simulink subsystem "BallAndPlate_transfer_function_model"  (R2024b)
settings: Solver=VariableStepAuto  StartTime=0.0  StopTime=10.0  RelTol=1e-3
libraries: cstblocks x2
settings Model: Creator=tshintai  LastModifiedBy=tshintai
settings OptimizationCC: ReuseModelBlockBuffer=off
settings DebuggingCC: UnconnectedInputMsg=warning  UnconnectedOutputMsg=warning  UnconnectedLineMsg=warning
settings ModelReferenceCC: EnableRefExpFcnMdlSchedulingChecks=on
settings RTWCC: GPUComputeCapability=3.5  DLArmComputeVersion=19.05

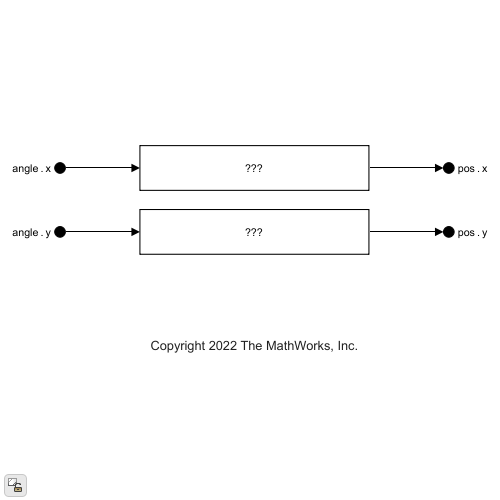
[thumbnail: Simulink's stored preview of the top-level diagram]
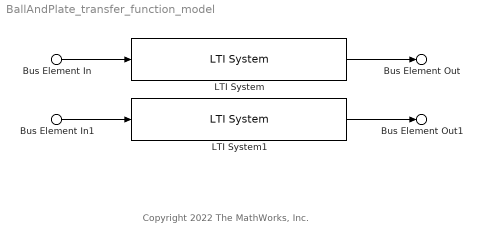
== system BallAndPlate_transfer_function_model ==
  note: Copyright 2022 The MathWorks, Inc.
  Bus Element In : Inport  PortName=angle  Element=x
  Bus Element In1 : Inport  PortName=angle  Element=y
  LTI System : cstblocks/LTI System  sys=estimated_BallAndPlate_transfer_function  IC=[]  PadeOrder=0
  LTI System1 : cstblocks/LTI System  sys=estimated_BallAndPlate_transfer_function  IC=[]  PadeOrder=0
  Bus Element Out : Outport  PortName=pos  Element=x
  Bus Element Out1 : Outport  PortName=pos  Element=y
  wires:
  Bus Element In1/1 -> LTI System1/1
  Bus Element In/1 -> LTI System/1
  LTI System/1 -> Bus Element Out/1
  LTI System1/1 -> Bus Element Out1/1
